simulink model "Fading_Rayleigh"  (R2022a)
settings: Solver=VariableStepAuto  StartTime=0.0  StopTime=simtime  FixedStep=1/2.45e6  RelTol=1e-3
values from neighbouring files (symbols this model uses):
  sSeed = 1    [savedata4k.m]
undefined symbols (not defined in the file or in its folder): doppler, No, W
libraries: commchan3 x2, commrandsrc3 x1
settings Model: Creator=roberto  LastModifiedBy=qanta
settings DebuggingCC: UnconnectedInputMsg=warning  UnconnectedOutputMsg=warning  UnconnectedLineMsg=warning
settings RTWCC: DLArmComputeVersion=19.05

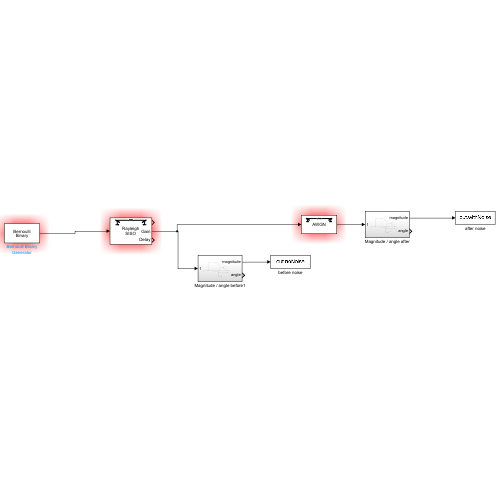
[thumbnail: Simulink's stored preview of the top-level diagram]
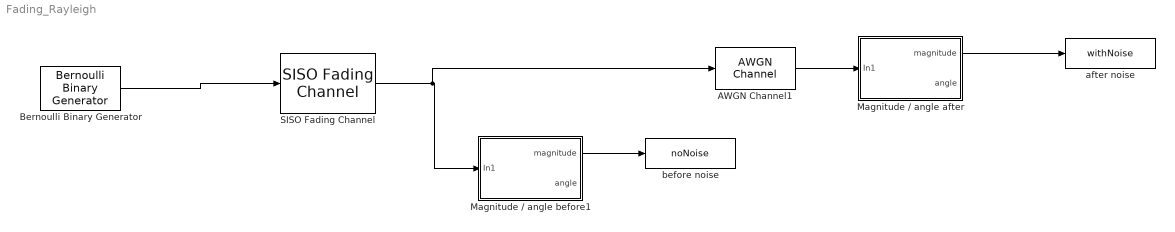
== system Fading_Rayleigh ==
  AWGN Channel1 : commchan3/AWGN Channel  InputProcessing=Columns as channels (frame based)  seed=67  noiseMode="Signal to noise ratio  (Eb/No)"  EbNodB=EbNo  EsNodB=10  SNRdB=7  bitsPerSym=1  Ps=1  Tsym=1/2e4  variance=No*W
  Bernoulli Binary Generator : commrandsrc3/Bernoulli Binary Generator  ProbabilityOfZero=0.5  SeedSource=Parameter  Seed=sSeed  SampleTime=1/2e4  SamplesPerFrame=1  OutputDataType=double  SimulateUsing=Interpreted execution
  Magnitude / angle after : Subsystem
  Magnitude / angle before1 : Subsystem
  SISO Fading Channel : commchan3/SISO Fading Channel  InheritSampleRate=off  SampleRate=sampleRate  PathDelays=rayDelay  AveragePathGains=rayGain  NormalizePathGains=off  FadingDistribution=Rayleigh  KFactor=3  DirectPathDopplerShift=0  DirectPathInitialPhase=0  MaximumDopplerShift=MDs  DopplerSpectrum=doppler('Jakes')  RandomStream=mt19937ar with seed  Seed=22  PathGainsOutputPort=on  ChannelFilterDelayOutputPort=on  SimulateUsing=Interpreted execution  Visualization=Off  PathsForDopplerDisplay=1  SamplesToDisplay=100%
  after noise : ToWorkspace  VariableName=withNoise  SampleTime=-1
  before noise : ToWorkspace  VariableName=noNoise  SampleTime=-1
  wires:
  Bernoulli Binary Generator/1 -> SISO Fading Channel/1
  AWGN Channel1/1 -> Magnitude / angle after/1(In1)
  Magnitude / angle after/1(magnitude) -> after noise/1
  SISO Fading Channel/2 -> AWGN Channel1/1, Magnitude / angle before1/1(In1)
  Magnitude / angle before1/1(magnitude) -> before noise/1

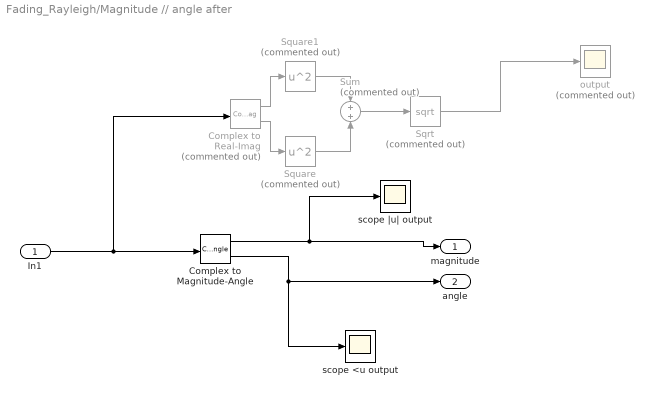
== system Fading_Rayleigh/Magnitude // angle after ==
  In1 : Inport
  Complex to Magnitude-Angle : ComplexToMagnitudeAngle
  Complex to Real-Imag : ComplexToRealImag  Commented=on
  Sqrt : Sqrt  Commented=on
  Square : Math  Commented=on  Operator=square
  Square1 : Math  Commented=on  Operator=square
  Sum : Sum  Commented=on
  output : Scope  Commented=on
  scope <u output : Scope
  scope |u| output : Scope
  magnitude : Outport
  angle : Outport  Port=2
  wires:
  Complex to Magnitude-Angle/1 -> scope |u| output/1, magnitude/1
  Square/1 -> Sum/2
  Complex to Real-Imag/1 -> Square1/1
  Square1/1 -> Sum/1
  Sum/1 -> Sqrt/1
  Complex to Real-Imag/2 -> Square/1
  In1/1 -> Complex to Real-Imag/1, Complex to Magnitude-Angle/1
  Complex to Magnitude-Angle/2 -> angle/1, scope <u output/1
  Sqrt/1 -> output/1

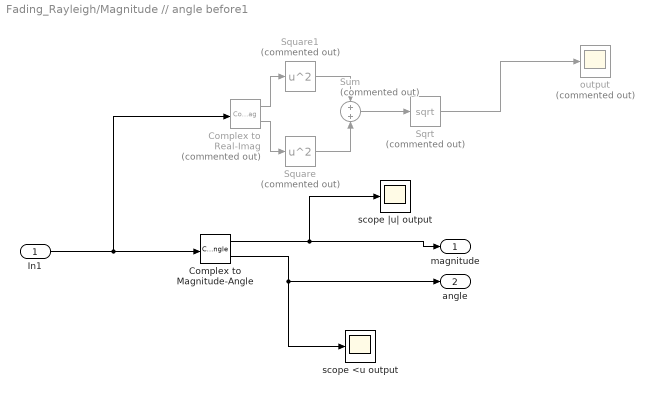
== system Fading_Rayleigh/Magnitude // angle before1 ==
  In1 : Inport
  Complex to Magnitude-Angle : ComplexToMagnitudeAngle
  Complex to Real-Imag : ComplexToRealImag  Commented=on
  Sqrt : Sqrt  Commented=on
  Square : Math  Commented=on  Operator=square
  Square1 : Math  Commented=on  Operator=square
  Sum : Sum  Commented=on
  output : Scope  Commented=on
  scope <u output : Scope
  scope |u| output : Scope
  magnitude : Outport
  angle : Outport  Port=2
  wires:
  Complex to Magnitude-Angle/1 -> scope |u| output/1, magnitude/1
  Square/1 -> Sum/2
  Complex to Real-Imag/1 -> Square1/1
  Square1/1 -> Sum/1
  Sum/1 -> Sqrt/1
  Complex to Real-Imag/2 -> Square/1
  In1/1 -> Complex to Real-Imag/1, Complex to Magnitude-Angle/1
  Complex to Magnitude-Angle/2 -> angle/1, scope <u output/1
  Sqrt/1 -> output/1
